simulink model "Tak11"  (R2021a)
settings: Solver=VariableStepAuto  StartTime=0.0  StopTime=5  RelTol=1e-3
values from neighbouring files (symbols this model uses):
  A = [5 3 ... (first row only)    [T_5.m]
  B = [0 ... (first row only)    [T_5.m]
  C = [5 0]    [T_5.m]
  D = 6    [T_5.m]
  G_overline = [0 -a_s(3) ... (first row only)    [T_5.m]
  Gamma_g = [0 1 ... (first row only)    [T_5.m]
  H_g = [1 0]    [T_5.m]
  K = -H/M    [T_5.m]
  L_overline = [0 ... (first row only)    [T_5.m]
  Lg = double([s.lg1 s.lg2])    [T_5.m]
  Mg_ov = double([sol.mg_ov1_1 sol.mg_ov1_2 ... (first row only)    [T_5.m]
  xi_0 = double([xi_1(0); xi_2(0)])    [T_5.m]
settings Model: Creator=fedor  LastModifiedBy=fedor

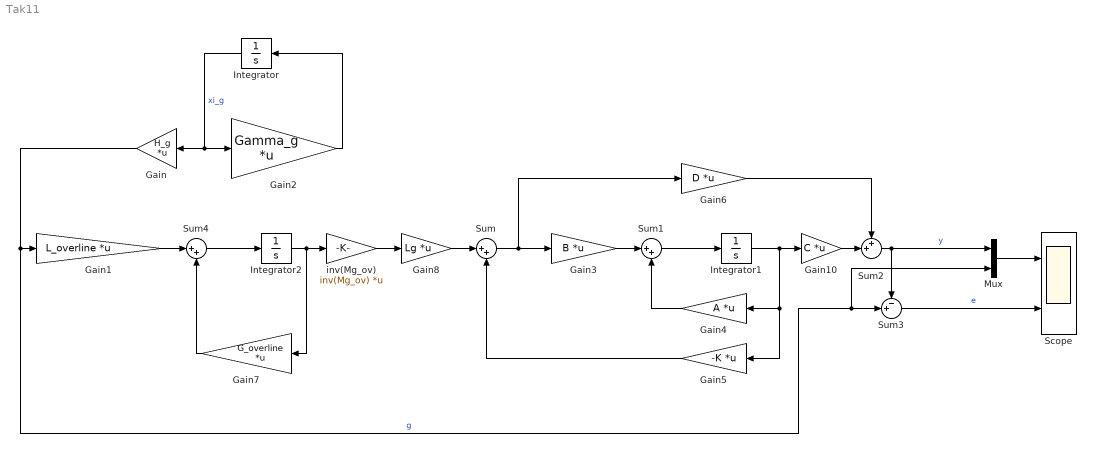
== system Tak11 ==
  Gain : Gain  Gain=H_g  Multiplication=Matrix(K*u)
  Gain1 : Gain  Gain=L_overline  Multiplication=Matrix(K*u)
  Gain10 : Gain  Gain=C  Multiplication=Matrix(K*u)
  Gain2 : Gain  Gain=Gamma_g  Multiplication=Matrix(K*u)
  Gain3 : Gain  Gain=B  Multiplication=Matrix(K*u)
  Gain4 : Gain  Gain=A  Multiplication=Matrix(K*u)
  Gain5 : Gain  Gain=-K  Multiplication=Matrix(K*u)
  Gain6 : Gain  Gain=D  Multiplication=Matrix(K*u)
  Gain7 : Gain  Gain=G_overline  Multiplication=Matrix(K*u)
  Gain8 : Gain  Gain=Lg  Multiplication=Matrix(K*u)
  Integrator : Integrator  InitialCondition=xi_0
  Integrator1 : Integrator
  Integrator2 : Integrator
  Mux : Mux  Inputs=2
  Scope : Scope  NumInputPorts=2
  Sum : Sum  Inputs=|++
  Sum1 : Sum  Inputs=|++
  Sum2 : Sum  Inputs=++|
  Sum3 : Sum  Inputs=-+|
  Sum4 : Sum  Inputs=|++
  inv(Mg_ov) : Gain  Gain=inv(Mg_ov)  Multiplication=Matrix(K*u)
  wires:
  Gain2/1 -> Integrator/1
  Integrator/1 -> Gain2/1, Gain/1  "xi_g"
  Sum/1 -> Gain6/1, Gain3/1
  Gain3/1 -> Sum1/1
  Sum1/1 -> Integrator1/1
  Gain5/1 -> Sum/2
  Gain4/1 -> Sum1/2
  Integrator1/1 -> Gain10/1, Gain4/1, Gain5/1
  Gain6/1 -> Sum2/1
  Sum2/1 -> Mux/1, Sum3/1  "y"
  Sum3/1 -> Scope/2  "e"
  Gain/1 -> Mux/2, Sum3/2, Gain1/1  "g"
  Sum4/1 -> Integrator2/1
  Gain7/1 -> Sum4/2
  Gain1/1 -> Sum4/1
  Gain8/1 -> Sum/1
  Integrator2/1 -> inv(Mg_ov)/1, Gain7/1
  inv(Mg_ov)/1 -> Gain8/1
  Gain10/1 -> Sum2/2
  Mux/1 -> Scope/1
